simulink model "PropulsionPlant_Vz_control"  (R2022b)
settings: Solver=ode15s  StartTime=0.0  StopTime=20  RelTol=1e-3
undefined symbols (not defined in the file or in its folder): Az, Bat, Bz, coeffs, env, ESC, fan, Gz, LookUp, motor, PX4, Ts, x0
libraries: slpidlib x2
settings Model: PauseTimes=1  Creator=User  LastModifiedBy=User

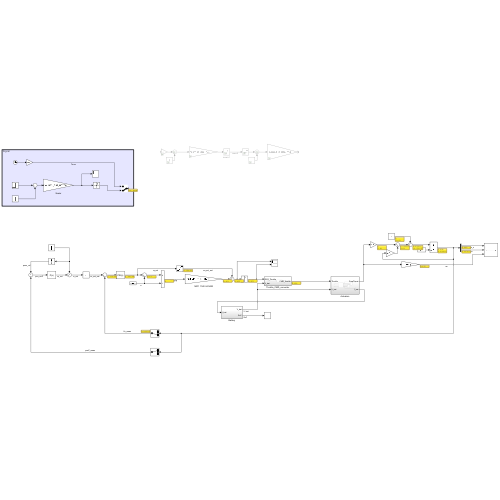
[thumbnail: Simulink's stored preview of the top-level diagram]
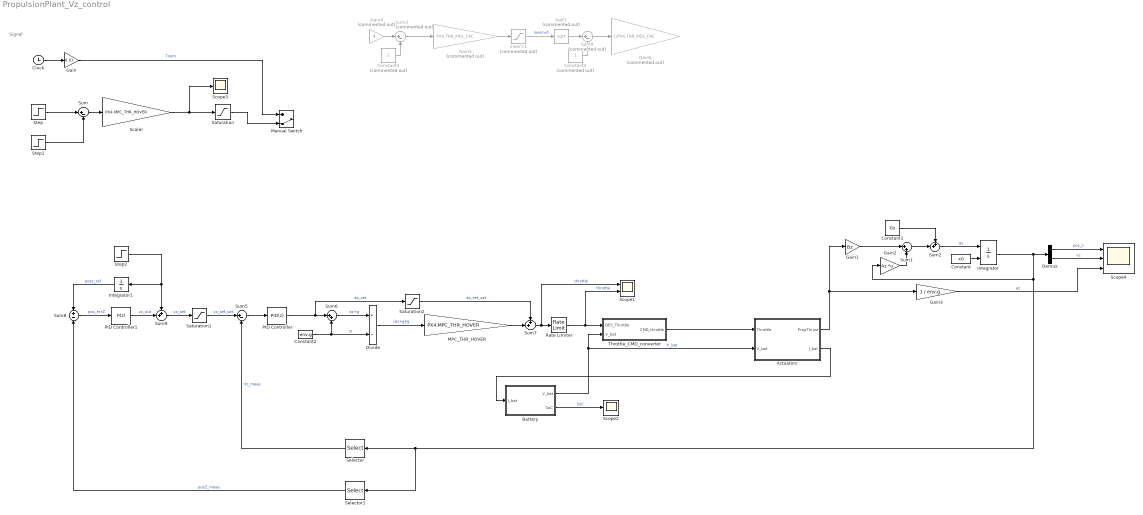
== system PropulsionPlant_Vz_control ==
  note: Signal
  Actuators : Subsystem
  Battery : Subsystem
  Clock : Clock
  Constant : Constant  Value=x0
  Constant1 : Constant  Value=Gz
  Constant2 : Constant  Value=env.g
  Constant3 : Constant  Commented=on
  Constant4 : Constant  Commented=on
  Demux : Demux  Outputs=2
  Divide : Product  Inputs=*/
  Gain : Gain  Gain=0.01
  Gain1 : Gain  Gain=Bz
  Gain2 : Gain  Gain=Az  Multiplication=Matrix(K*u)
  Gain3 : Gain  Gain=1 / env.g
  Gain4 : Gain  Commented=on  Gain=4
  Gain5 : Gain  Commented=on  Gain=PX4.THR_MDL_FAC
  Gain6 : Gain  Commented=on  Gain=1/PX4.THR_MDL_FAC
  Integrator : Integrator  InitialConditionSource=external
  Integrator1 : Integrator
  MPC_THR_HOVER : Gain  Gain=PX4.MPC_THR_HOVER
  Manual Switch : ManualSwitch  CurrentSetting=0
  PID Controller : slpidlib/PID Controller  Controller=PID  Form=Parallel  TimeDomain=Discrete-time  UseExternalTs=off  SampleTime=Ts  IntegratorMethod=Forward Euler  FilterMethod=Forward Euler  ControllerParametersSource=internal  P=0.5  I=0  UseKiTs=off  D=0  N=100  UseFilter=on  TunerSelectOption=Transfer Function Based (PID Tuner App)  InitialConditionSource=internal  InitialConditionForIntegrator=0  InitialConditionForFilter=0  DifferentiatorICPrevScaledInput=0  ExternalReset=none  TrackingMode=off  Kt=1  LimitOutput=off  SatLimitsSource=internal  UpperSaturationLimit=inf  LowerSaturationLimit=-inf  LinearizeAsGain=on  AntiWindupMode=none  Kb=1  LimitIntegrator=off  UpperIntegratorSaturationLimit=inf  LowerIntegratorSaturationLimit=-inf  POutMin=[]  POutMax=[]  IOutMin=[]  IOutMax=[]  DOutMin=[]  DOutMax=[]  NOutMin=[]  NOutMax=[]  SumOutMin=[]  SumOutMax=[]  SaturationOutMin=[]  SaturationOutMax=[]  PParamMin=[]  PParamMax=[]  IParamMin=[]  IParamMax=[]  DParamMin=[]  DParamMax=[]  NParamMin=[]  NParamMax=[]  KbParamMin=[]  KbParamMax=[]  KtParamMin=[]  KtParamMax=[]  KbOutMin=[]  KbOutMax=[]  KtOutMin=[]  KtOutMax=[]  IntegratorOutMin=[]  IntegratorOutMax=[]  FilterOutMin=[]  FilterOutMax=[]  SumI1OutMin=[]  SumI1OutMax=[]  SumI2OutMin=[]  SumI2OutMax=[]  SumI3OutMin=[]  SumI3OutMax=[]  SumI4OutMin=[]  SumI4OutMax=[]  SumDOutMin=[]  SumDOutMax=[]  DifferentiatorOutMin=[]  DifferentiatorOutMax=[]  FilterDiffOutCoefMin=[]  FilterDiffOutCoefMax=[]  ReciprocalOutMin=[]  ReciprocalOutMax=[]  SumDenOutMin=[]  SumDenOutMax=[]  SumNumOutMin=[]  SumNumOutMax=[]  DivideOutMin=[]  DivideOutMax=[]  UdiffTsProdOutMin=[]  UdiffTsProdOutMax=[]  NTsProdOutMin=[]  NTsProdOutMax=[]  UintegralTsProdOutMin=[]  UintegralTsProdOutMax=[]  UngainTsProdOutMin=[]  UngainTsProdOutMax=[]  ClampingZeroOutDataTypeStr=Inherit: Inherit via back propagation  ClampingZeroOutMin=[]  ClampingZeroOutMax=[]  FilterDenConstantOutDataTypeStr=Inherit: Inherit via back propagation  FilterDenConstantOutMin=[]  FilterDenConstantOutMax=[]  PCopyOutDataTypeStr=Inherit: Inherit via back propagation  PCopyOutMin=[]  PCopyOutMax=[]  NCopyOutDataTypeStr=Inherit: Inherit via back propagation  NCopyOutMin=[]  NCopyOutMax=[]  IntegratorContinuousStateAttributes=''  IntegratorStateMustResolveToSignalObject=off  IntegratorRTWStateStorageClass=Auto  FilterContinuousStateAttributes=''  FilterStateMustResolveToSignalObject=off  FilterRTWStateStorageClass=Auto  ParallelPVariant=InternalParameters  IdealPVariant=Disabled  IVariant=InternalParameters  DVariant=InternalParameters  IntegratorVariant=Discrete  SatVariant=Disabled  AWVariant=Passthrough  PCopyVariant=Disabled  TRVariant=Disabled  FdbkBlocksVariant=Forward  IdealPFdbkVariant=Disabled  SatFdbkVariant=Disabled  DerivativeFilterVariant=ForwardEulerFilter  NVariant=InternalParameters  NCopyVariant=Disabled  FilterICVariant=InternalICsFilter  IntegratorICVariant=InternalICs  ExternalResetVariant=Disabled  TRSumVariant=Passthrough  SumFdbkVariant=Disabled  SumVariant=Sum_PID  TsampFilterVariant=InternalTs  TsampNgainVariant=Passthrough  TsampIntegralVariant=Passthrough  ExternalSaturationOutDataTypeStr=Inherit: Same as second input
  PID Controller1 : slpidlib/PID Controller  Controller=P  Form=Parallel  TimeDomain=Discrete-time  UseExternalTs=off  SampleTime=Ts  IntegratorMethod=Forward Euler  FilterMethod=Forward Euler  ControllerParametersSource=internal  P=0.1  I=0  UseKiTs=off  D=0  N=100  UseFilter=on  TunerSelectOption=Transfer Function Based (PID Tuner App)  InitialConditionSource=internal  InitialConditionForIntegrator=0  InitialConditionForFilter=0  DifferentiatorICPrevScaledInput=0  ExternalReset=none  TrackingMode=off  Kt=1  LimitOutput=off  SatLimitsSource=internal  UpperSaturationLimit=inf  LowerSaturationLimit=-inf  LinearizeAsGain=on  AntiWindupMode=none  Kb=1  LimitIntegrator=off  UpperIntegratorSaturationLimit=inf  LowerIntegratorSaturationLimit=-inf  POutMin=[]  POutMax=[]  IOutMin=[]  IOutMax=[]  DOutMin=[]  DOutMax=[]  NOutMin=[]  NOutMax=[]  SumOutMin=[]  SumOutMax=[]  SaturationOutMin=[]  SaturationOutMax=[]  PParamMin=[]  PParamMax=[]  IParamMin=[]  IParamMax=[]  DParamMin=[]  DParamMax=[]  NParamMin=[]  NParamMax=[]  KbParamMin=[]  KbParamMax=[]  KtParamMin=[]  KtParamMax=[]  KbOutMin=[]  KbOutMax=[]  KtOutMin=[]  KtOutMax=[]  IntegratorOutMin=[]  IntegratorOutMax=[]  FilterOutMin=[]  FilterOutMax=[]  SumI1OutMin=[]  SumI1OutMax=[]  SumI2OutMin=[]  SumI2OutMax=[]  SumI3OutMin=[]  SumI3OutMax=[]  SumI4OutMin=[]  SumI4OutMax=[]  SumDOutMin=[]  SumDOutMax=[]  DifferentiatorOutMin=[]  DifferentiatorOutMax=[]  FilterDiffOutCoefMin=[]  FilterDiffOutCoefMax=[]  ReciprocalOutMin=[]  ReciprocalOutMax=[]  SumDenOutMin=[]  SumDenOutMax=[]  SumNumOutMin=[]  SumNumOutMax=[]  DivideOutMin=[]  DivideOutMax=[]  UdiffTsProdOutMin=[]  UdiffTsProdOutMax=[]  NTsProdOutMin=[]  NTsProdOutMax=[]  UintegralTsProdOutMin=[]  UintegralTsProdOutMax=[]  UngainTsProdOutMin=[]  UngainTsProdOutMax=[]  ClampingZeroOutDataTypeStr=Inherit: Inherit via back propagation  ClampingZeroOutMin=[]  ClampingZeroOutMax=[]  FilterDenConstantOutDataTypeStr=Inherit: Inherit via back propagation  FilterDenConstantOutMin=[]  FilterDenConstantOutMax=[]  PCopyOutDataTypeStr=Inherit: Inherit via back propagation  PCopyOutMin=[]  PCopyOutMax=[]  NCopyOutDataTypeStr=Inherit: Inherit via back propagation  NCopyOutMin=[]  NCopyOutMax=[]  IntegratorContinuousStateAttributes=''  IntegratorStateMustResolveToSignalObject=off  IntegratorRTWStateStorageClass=Auto  FilterContinuousStateAttributes=''  FilterStateMustResolveToSignalObject=off  FilterRTWStateStorageClass=Auto  ParallelPVariant=InternalParameters  IdealPVariant=Disabled  IVariant=Disabled  DVariant=Disabled  IntegratorVariant=Disabled  SatVariant=Disabled  AWVariant=Disabled  PCopyVariant=Disabled  TRVariant=Disabled  FdbkBlocksVariant=Forward  IdealPFdbkVariant=Disabled  SatFdbkVariant=Disabled  DerivativeFilterVariant=Disabled  NVariant=Disabled  NCopyVariant=Disabled_SignalSpec  FilterICVariant=Disabled  IntegratorICVariant=Disabled  ExternalResetVariant=Disabled  TRSumVariant=Passthrough  SumFdbkVariant=Disabled  SumVariant=Passthrough_P  TsampFilterVariant=InternalTs  TsampNgainVariant=Passthrough  TsampIntegralVariant=Disabled_SignalSpec  ExternalSaturationOutDataTypeStr=Inherit: Same as second input
  Rate Limiter : RateLimiter  RisingSlewLimit=PX4.MOT_SLEW_MAX  FallingSlewLimit=-PX4.MOT_SLEW_MAX  SampleTimeMode=inherited
  Saturation : Saturate  UpperLimit=PX4.MPC_THR_MAX  LowerLimit=PX4.MPC_THR_MIN
  Saturation1 : Saturate  UpperLimit=PX4.MPC_Z_VEL_MAX_UP  LowerLimit=PX4.MPC_Z_VEL_MAX_DN
  Saturation2 : Saturate  UpperLimit=PX4.MPC_ACC_UP_MAX  LowerLimit=PX4.MPC_ACC_DOWN_MAX
  Scaler : Gain  Gain=PX4.MPC_THR_HOVER
  Scope1 : Scope  NumInputPorts=2
  Scope2 : Scope
  Scope3 : Scope
  Scope4 : Scope  NumInputPorts=3
  Selector : Selector  InputPortWidth=2  IndexOptions=Index vector (dialog)  Indices=[ 2]  OutputSizes=1
  Selector1 : Selector  InputPortWidth=2  IndexOptions=Index vector (dialog)  Indices=[1]  OutputSizes=1
  Sqrt1 : Sqrt  Commented=on
  Step : Step  Time=0  Before=1  SampleTime=0
  Step1 : Step  Time=100  SampleTime=0
  Step2 : Step  Before=1  After=0  SampleTime=Ts
  Sum : Sum  Inputs=|+-
  Sum1 : Sum  Inputs=|++
  Sum2 : Sum  Inputs=++|
  Sum3 : Sum  Commented=on  Inputs=|+-
  Sum4 : Sum  Commented=on  Inputs=|+-
  Sum5 : Sum  Inputs=|+-
  Sum6 : Sum  Inputs=|++
  Sum7 : Sum  Inputs=++|
  Sum8 : Sum  Inputs=+|-
  Sum9 : Sum  Inputs=++|
  Throttle_CMD_converter : Subsystem
  inner>1 : Saturate  Commented=on  UpperLimit=1e10  LowerLimit=0
  wires:
  Battery/1(V_bat) -> Throttle_CMD_converter/2(V_bat), Actuators/2(V_bat)  "V_bat"
  Scaler/1 -> Scope3/1, Saturation/1
  Battery/2(SoC) -> Scope2/1  "SoC"
  Step/1 -> Sum/1
  Step1/1 -> Sum/2
  Sum/1 -> Scaler/1
  Saturation/1 -> Manual Switch/2
  Clock/1 -> Gain/1
  Sum4/1 -> Gain6/1
  Constant4/1 -> Sum4/2
  inner>1/1 -> Sqrt1/1  "inner>0"
  Gain4/1 -> Sum3/1
  Constant3/1 -> Sum3/2
  Sqrt1/1 -> Sum4/1
  Sum3/1 -> Gain5/1
  Gain5/1 -> inner>1/1
  Gain/1 -> Manual Switch/1  "Tnom"
  Sum2/1 -> Integrator/1  "az"
  Constant/1 -> Integrator/2
  Gain2/1 -> Sum1/2
  Gain1/1 -> Sum1/1
  Integrator/1 -> Gain2/1, Selector1/1, Selector/1, Demux/1
  Constant1/1 -> Sum2/1
  Sum1/1 -> Sum2/2
  Demux/1 -> Scope4/1  "pos_z"
  Demux/2 -> Scope4/2  "vz"
  Gain3/1 -> Scope4/3  "az"
  Sum5/1 -> PID Controller/1
  Selector/1 -> Sum5/2  "Vz_meas"
  PID Controller/1 -> Saturation2/1, Sum6/1  "az_set"
  Constant2/1 -> Sum6/2, Divide/2  "g"
  Sum6/1 -> Divide/1  "az+g"
  Divide/1 -> MPC_THR_HOVER/1  "(az+g)/g"
  Rate Limiter/1 -> Scope1/2, Throttle_CMD_converter/1(DES_Throttle)  "throttle"
  Integrator1/1 -> Sum8/1  "posz_ref"
  Sum8/1 -> PID Controller1/1  "pos_errZ"
  PID Controller1/1 -> Sum9/2  "vz_out"
  Step2/1 -> Integrator1/1, Sum9/1
  Selector1/1 -> Sum8/2  "posZ_meas"
  Sum9/1 -> Saturation1/1  "vz_set"
  Saturation1/1 -> Sum5/1  "vz_set_sat"
  Saturation2/1 -> Sum7/1  "az_set_sat"
  MPC_THR_HOVER/1 -> Sum7/2
  Sum7/1 -> Scope1/1, Rate Limiter/1  "throttle"
  Actuators/1(PropThrust) -> Gain1/1, Gain3/1
  Throttle_CMD_converter/1(CMD_throttle) -> Actuators/1(Throttle)
  Actuators/2(I_bat) -> Battery/1(I_bat)

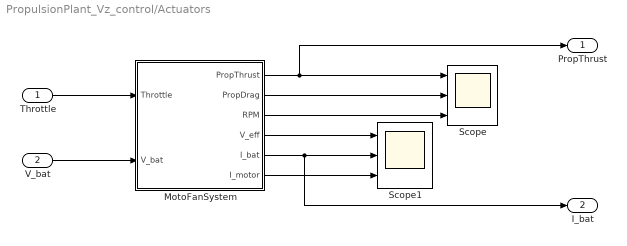
== system PropulsionPlant_Vz_control/Actuators ==
  Throttle : Inport
  V_bat : Inport  Port=2
  MotoFanSystem : Subsystem
  Scope : Scope  NumInputPorts=3
  Scope1 : Scope  NumInputPorts=3
  PropThrust : Outport
  I_bat : Outport  Port=2
  wires:
  MotoFanSystem/1(PropThrust) -> PropThrust/1, Scope/1
  V_bat/1 -> MotoFanSystem/2(V_bat)
  MotoFanSystem/3(RPM) -> Scope/3
  MotoFanSystem/6(I_motor) -> Scope1/3
  MotoFanSystem/4(V_eff) -> Scope1/1
  MotoFanSystem/5(I_bat) -> I_bat/1, Scope1/2
  MotoFanSystem/2(PropDrag) -> Scope/2
  Throttle/1 -> MotoFanSystem/1(Throttle)

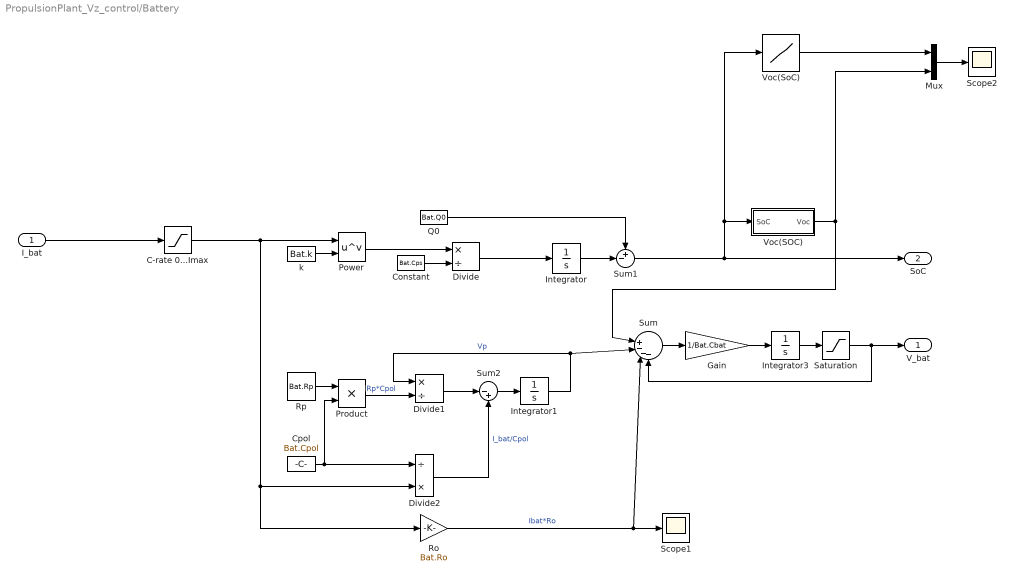
== system PropulsionPlant_Vz_control/Battery ==
  I_bat : Inport
  C-rate 0...Imax : Saturate  UpperLimit=Bat.Imax  LowerLimit=ESC.I_idle
  Constant : Constant  Value=Bat.Cps
  Cpol : Constant  Value=Bat.Cpol
  Divide : Product  Inputs=*/
  Divide1 : Product  Inputs=*/
  Divide2 : Product  Inputs=/*
  Gain : Gain  Gain=1/Bat.Cbat
  Integrator : Integrator
  Integrator1 : Integrator
  Integrator3 : Integrator  InitialCondition=Bat.Vcell*Bat.ncell
  Mux : Mux  Inputs=2
  Power : Math  Operator=pow
  Product : Product
  Q0 : Constant  Value=Bat.Q0
  Ro : Gain  Gain=Bat.Ro
  Rp : Constant  Value=Bat.Rp
  Saturation : Saturate  UpperLimit=Bat.Voc  LowerLimit=0
  Scope1 : Scope
  Scope2 : Scope
  Sum : Sum  Inputs=||+---
  Sum1 : Sum  Inputs=+-|
  Sum2 : Sum  Inputs=|-+
  Voc(SOC) : Subsystem
  Voc(SoC) : Lookup_n-D  NumberOfTableDimensions=1  BreakpointsForDimension1=LookUp.SoC  Table=LookUp.Volts  InternalRulePriority=Speed  RndMeth=Simplest
  k : Constant  Value=Bat.k
  V_bat : Outport
  SoC : Outport  Port=2
  wires:
  Integrator1/1 -> Divide1/1, Sum/2  "Vp"
  Sum2/1 -> Integrator1/1
  Product/1 -> Divide1/2  "Rp*Cpol"
  Q0/1 -> Sum1/1
  Cpol/1 -> Divide2/1, Product/2
  Voc(SoC)/1 -> Mux/1
  Rp/1 -> Product/1
  Power/1 -> Divide/1
  Constant/1 -> Divide/2
  k/1 -> Power/2
  Sum/1 -> Gain/1
  I_bat/1 -> C-rate 0...Imax/1
  Integrator/1 -> Sum1/2
  Divide1/1 -> Sum2/1
  Divide2/1 -> Sum2/2  "I_bat/Cpol"
  Ro/1 -> Sum/3, Scope1/1  "Ibat*Ro"
  Divide/1 -> Integrator/1
  C-rate 0...Imax/1 -> Ro/1, Divide2/2, Power/1
  Integrator3/1 -> Saturation/1
  Gain/1 -> Integrator3/1
  Sum1/1 -> Voc(SoC)/1, Voc(SOC)/1(SoC), SoC/1
  Saturation/1 -> V_bat/1, Sum/4
  Voc(SOC)/1(Voc) -> Sum/1, Mux/2
  Mux/1 -> Scope2/1

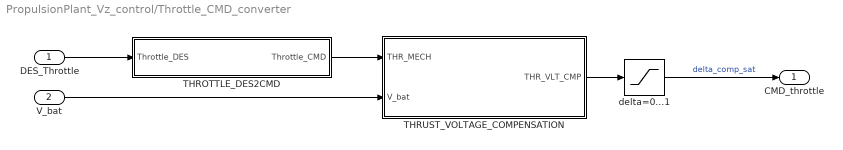
== system PropulsionPlant_Vz_control/Throttle_CMD_converter ==
  DES_Throttle : Inport
  V_bat : Inport  Port=2
  THROTTLE_DES2CMD : Subsystem
  THRUST_VOLTAGE_COMPENSATION : Subsystem
  delta=0...1 : Saturate  UpperLimit=1  LowerLimit=0
  CMD_throttle : Outport
  wires:
  THROTTLE_DES2CMD/1(Throttle_CMD) -> THRUST_VOLTAGE_COMPENSATION/1(THR_MECH)
  V_bat/1 -> THRUST_VOLTAGE_COMPENSATION/2(V_bat)
  delta=0...1/1 -> CMD_throttle/1  "delta_comp_sat"
  THRUST_VOLTAGE_COMPENSATION/1(THR_VLT_CMP) -> delta=0...1/1
  DES_Throttle/1 -> THROTTLE_DES2CMD/1(Throttle_DES)

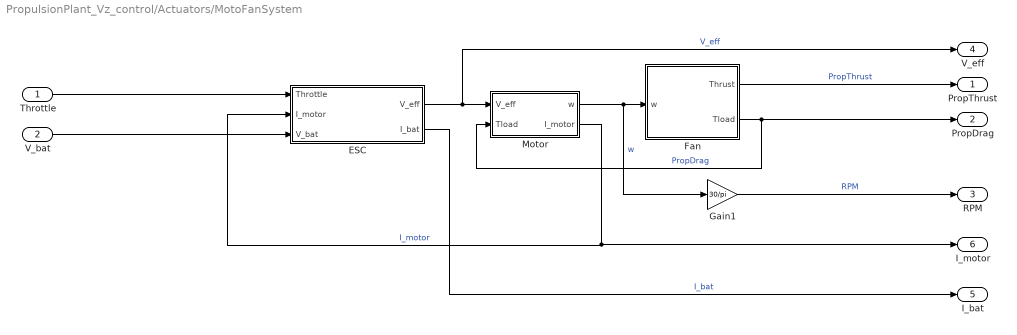
== system PropulsionPlant_Vz_control/Actuators/MotoFanSystem ==
  Throttle : Inport
  V_bat : Inport  Port=2
  ESC : Subsystem
  Fan : Subsystem
  Gain1 : Gain  Gain=30/pi
  Motor : Subsystem
  PropThrust : Outport
  PropDrag : Outport  Port=2
  RPM : Outport  Port=3
  V_eff : Outport  Port=4
  I_bat : Outport  Port=5
  I_motor : Outport  Port=6
  wires:
  ESC/2(I_bat) -> I_bat/1  "I_bat"
  Motor/2(I_motor) -> ESC/2(I_motor), I_motor/1  "I_motor"
  Motor/1(w) -> Gain1/1, Fan/1(w)  "w"
  ESC/1(V_eff) -> V_eff/1, Motor/1(V_eff)  "V_eff"
  Gain1/1 -> RPM/1  "RPM"
  Fan/2(Tload) -> Motor/2(Tload), PropDrag/1  "PropDrag"
  Throttle/1 -> ESC/1(Throttle)
  Fan/1(Thrust) -> PropThrust/1  "PropThrust"
  V_bat/1 -> ESC/3(V_bat)

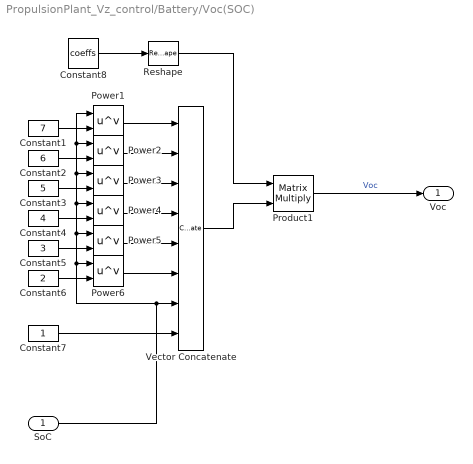
== system PropulsionPlant_Vz_control/Battery/Voc(SOC) ==
  SoC : Inport
  Constant1 : Constant  Value=7
  Constant2 : Constant  Value=6
  Constant3 : Constant  Value=5
  Constant4 : Constant  Value=4
  Constant5 : Constant  Value=3
  Constant6 : Constant  Value=2
  Constant7 : Constant
  Constant8 : Constant  Value=coeffs
  Power{1..6} (6 alike) : Math  Operator=pow
  Product1 : Product  Multiplication=Matrix(*)
  Reshape : Reshape  OutputDimensionality=Row vector (2-D)
  Vector Concatenate : Concatenate  NumInputs=8
  Voc : Outport
  wires:
  Power3/1 -> Vector Concatenate/3
  Power4/1 -> Vector Concatenate/4
  Constant8/1 -> Reshape/1
  Power6/1 -> Vector Concatenate/6
  Power1/1 -> Vector Concatenate/1
  Constant5/1 -> Power5/2
  SoC/1 -> Vector Concatenate/7, Power1/1, Power2/1, Power3/1, Power4/1, Power5/1, Power6/1
  Constant3/1 -> Power3/2
  Power5/1 -> Vector Concatenate/5
  Power2/1 -> Vector Concatenate/2
  Constant7/1 -> Vector Concatenate/8
  Constant2/1 -> Power2/2
  Constant6/1 -> Power6/2
  Constant1/1 -> Power1/2
  Constant4/1 -> Power4/2
  Reshape/1 -> Product1/1
  Product1/1 -> Voc/1  "Voc"
  Vector Concatenate/1 -> Product1/2

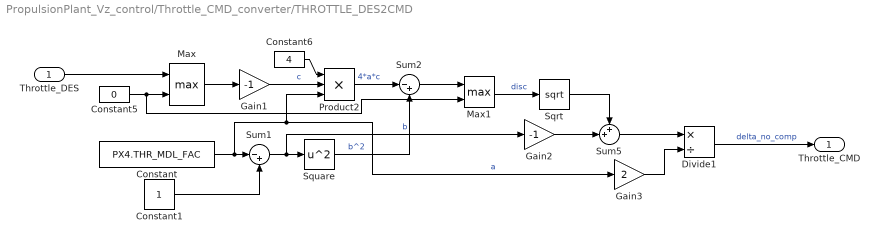
== system PropulsionPlant_Vz_control/Throttle_CMD_converter/THROTTLE_DES2CMD ==
  Throttle_DES : Inport
  Constant : Constant  Value=PX4.THR_MDL_FAC
  Constant1 : Constant
  Constant5 : Constant  Value=0
  Constant6 : Constant  Value=4
  Divide1 : Product  Inputs=*/
  Gain1 : Gain  Gain=-1
  Gain2 : Gain  Gain=-1
  Gain3 : Gain  Gain=2
  Max : MinMax  Function=max  Inputs=2
  Max1 : MinMax  Function=max  Inputs=2
  Product2 : Product  Inputs=3
  Sqrt : Sqrt
  Square : Math  Operator=square
  Sum1 : Sum  Inputs=|-+
  Sum2 : Sum  Inputs=|-+
  Sum5 : Sum  Inputs=++|
  Throttle_CMD : Outport
  wires:
  Max1/1 -> Sqrt/1  "disc"
  Max/1 -> Gain1/1
  Constant/1 -> Gain3/1, Product2/3, Sum1/1  "a"
  Gain3/1 -> Divide1/2
  Constant1/1 -> Sum1/2
  Sqrt/1 -> Sum5/1
  Sum5/1 -> Divide1/1
  Constant6/1 -> Product2/1
  Constant5/1 -> Max1/2, Max/2
  Sum1/1 -> Gain2/1, Square/1  "b"
  Sum2/1 -> Max1/1
  Gain1/1 -> Product2/2  "c"
  Gain2/1 -> Sum5/2
  Square/1 -> Sum2/2  "b^2"
  Product2/1 -> Sum2/1  "4*a*c"
  Throttle_DES/1 -> Max/1
  Divide1/1 -> Throttle_CMD/1  "delta_no_comp"

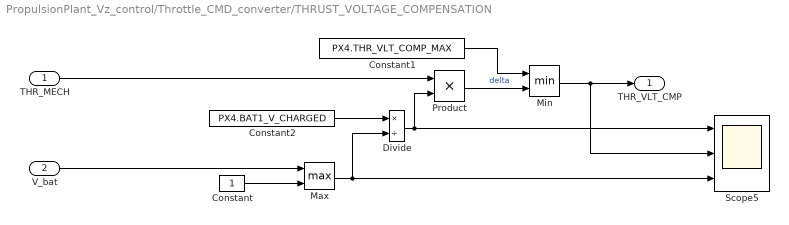
== system PropulsionPlant_Vz_control/Throttle_CMD_converter/THRUST_VOLTAGE_COMPENSATION ==
  THR_MECH : Inport
  V_bat : Inport  Port=2
  Constant : Constant
  Constant1 : Constant  Value=PX4.THR_VLT_COMP_MAX
  Constant2 : Constant  Value=PX4.BAT1_V_CHARGED
  Divide : Product  Inputs=*/
  Max : MinMax  Function=max  Inputs=2
  Min : MinMax  Inputs=2
  Product : Product
  Scope5 : Scope  NumInputPorts=3
  THR_VLT_CMP : Outport
  wires:
  THR_MECH/1 -> Product/1
  Max/1 -> Divide/2, Scope5/3
  Constant2/1 -> Divide/1
  V_bat/1 -> Max/1
  Divide/1 -> Product/2, Scope5/1
  Product/1 -> Min/2  "delta"
  Constant/1 -> Max/2
  Min/1 -> Scope5/2, THR_VLT_CMP/1
  Constant1/1 -> Min/1

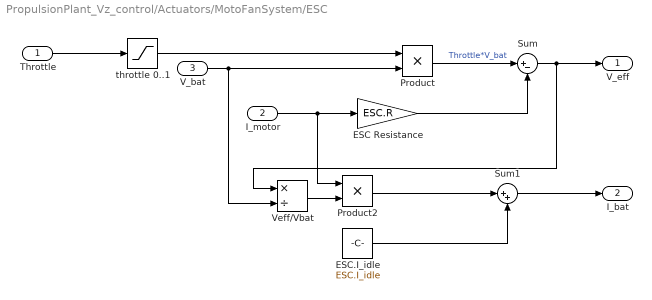
== system PropulsionPlant_Vz_control/Actuators/MotoFanSystem/ESC ==
  Throttle : Inport
  I_motor : Inport  Port=2
  V_bat : Inport  Port=3
  ESC Resistance : Gain  Gain=ESC.R
  ESC.I_idle : Constant  Value=ESC.I_idle
  Product : Product
  Product2 : Product
  Sum : Sum  Inputs=|+-
  Sum1 : Sum  Inputs=|++
  Veff/Vbat : Product  Inputs=*/
  throttle 0..1 : Saturate  UpperLimit=1  LowerLimit=0
  V_eff : Outport
  I_bat : Outport  Port=2
  wires:
  Throttle/1 -> throttle 0..1/1
  V_bat/1 -> Product/2, Veff/Vbat/2
  Product/1 -> Sum/1  "Throttle*V_bat"
  Sum1/1 -> I_bat/1
  ESC Resistance/1 -> Sum/2
  Sum/1 -> V_eff/1, Veff/Vbat/1
  I_motor/1 -> ESC Resistance/1, Product2/1
  Veff/Vbat/1 -> Product2/2
  Product2/1 -> Sum1/1
  ESC.I_idle/1 -> Sum1/2
  throttle 0..1/1 -> Product/1

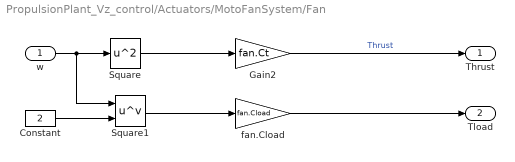
== system PropulsionPlant_Vz_control/Actuators/MotoFanSystem/Fan ==
  w : Inport
  Constant : Constant  Value=2
  Gain2 : Gain  Gain=fan.Ct
  Square : Math  Operator=square
  Square1 : Math  Operator=pow
  fan.Cload : Gain  Gain=fan.Cload
  Thrust : Outport
  Tload : Outport  Port=2
  wires:
  Square/1 -> Gain2/1
  Gain2/1 -> Thrust/1  "Thrust"
  w/1 -> Square1/1, Square/1
  Constant/1 -> Square1/2
  Square1/1 -> fan.Cload/1
  fan.Cload/1 -> Tload/1

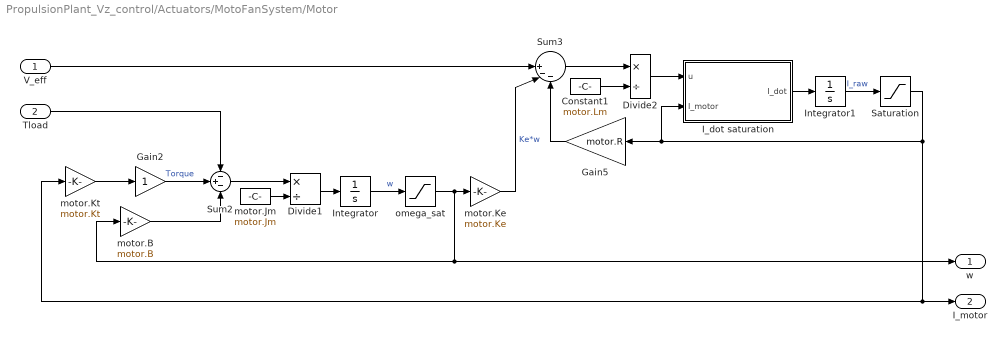
== system PropulsionPlant_Vz_control/Actuators/MotoFanSystem/Motor ==
  V_eff : Inport
  Tload : Inport  Port=2
  Constant1 : Constant  Value=motor.Lm
  Divide1 : Product  Inputs=*/
  Divide2 : Product  Inputs=*/
  Gain2 : Gain
  Gain5 : Gain  Gain=motor.R
  I_dot saturation : MATLAB Function  TreatAsAtomicUnit=on
  Integrator : Integrator
  Integrator1 : Integrator
  Saturation : Saturate  UpperLimit=motor.Imax  LowerLimit=-motor.Imax
  Sum2 : Sum  Inputs=-+-
  Sum3 : Sum  Inputs=||+--
  motor.B : Gain  Gain=motor.B
  motor.Jm : Constant  Value=motor.Jm
  motor.Ke : Gain  Gain=motor.Ke
  motor.Kt : Gain  Gain=motor.Kt
  omega_sat : Saturate  UpperLimit=motor.maxFreq  LowerLimit=0
  w : Outport
  I_motor : Outport  Port=2
  wires:
  motor.Jm/1 -> Divide1/2
  Divide1/1 -> Integrator/1
  motor.Kt/1 -> Gain2/1
  Integrator/1 -> omega_sat/1  "w"
  Constant1/1 -> Divide2/2
  motor.Ke/1 -> Sum3/2  "Ke*w"
  Integrator1/1 -> Saturation/1  "I_raw"
  V_eff/1 -> Sum3/1
  Gain2/1 -> Sum2/2  "Torque"
  Sum2/1 -> Divide1/1
  Tload/1 -> Sum2/1
  motor.B/1 -> Sum2/3
  Sum3/1 -> Divide2/1
  Gain5/1 -> Sum3/3
  Saturation/1 -> I_dot saturation/2(I_motor), Gain5/1, motor.Kt/1, I_motor/1
  Divide2/1 -> I_dot saturation/1(u)
  I_dot saturation/1(I_dot) -> Integrator1/1
  omega_sat/1 -> motor.B/1, w/1, motor.Ke/1

== matlab function PropulsionPlant_Vz_control/Actuators/MotoFanSystem/Motor/I_dot saturation ==
  data: u input; I_dot output; I_motor input
function I_dot = Idot(u, I_motor)

% parameters (define as mask parameters or globals)
I_max = 120;     % example
u_max = 1e6;     % A/s, numerical safety limit

% guard against NaN / Inf
if ~isfinite(u)
    I_dot = 0;
    return;
end

% limit derivative (ESC bandwidth / numerical safety)
u = max(min(u, u_max), -u_max);

% saturation detection (NOT at zero!)
sat = abs(I_motor) >= I_max;

% pushing further only if current is nonzero
push = (I_motor ~= 0) && (sign(u) == sign(I_motor));

if sat && push
    I_dot = 0;
else
    I_dot = u;
end
